simulink model "send_mmf"  (R2016a)
settings: Solver=FixedStepAuto  StartTime=0.0  StopTime=10.0  RelTol=1e-3
libraries: simulink x1, dspsigops x1, dspnetwork x1
settings Model: Creator=Florian Wachter  LastModifiedBy=Florian

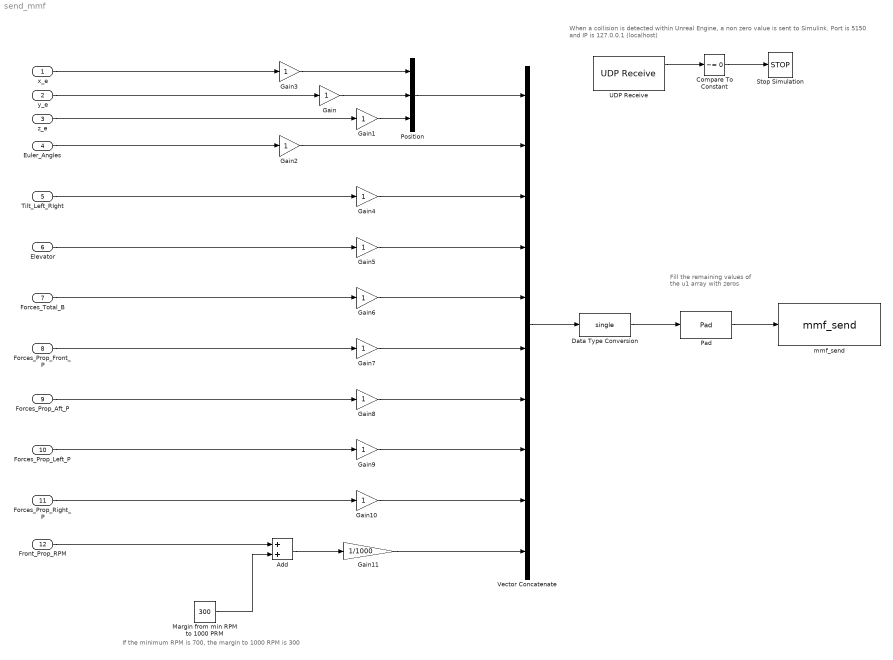
== system send_mmf ==
  note: If the minimum RPM is 700, the margin to 1000 RPM is 300
  note: Fill the remaining values of the u1 array with zeros
  note: When a collision is detected within Unreal Engine, a non zero value is sent to Simulink. Port is 5150 and IP is 127.0.0.1 (localhost)
  x_e : Inport
  y_e : Inport  Port=2
  z_e : Inport  Port=3
  Euler_Angles : Inport  Port=4
  Tilt_Left_RIght : Inport  Port=5
  Elevator : Inport  Port=6
  Forces_Total_B : Inport  Port=7
  Forces_Prop_Front_P : Inport  Port=8
  Forces_Prop_Aft_P : Inport  Port=9
  Forces_Prop_Left_P : Inport  Port=10
  Forces_Prop_Right_P : Inport  Port=11
  Front_Prop_RPM : Inport  Port=12
  Add : Sum
  Compare To Constant : simulink/Logic and Bit Operations/Compare To Constant  relop=~=  const=0  OutDataTypeStr=boolean
  Data Type Conversion : DataTypeConversion  OutMax=[100]  OutDataTypeStr=single
  Gain{,1..10} (11 alike) : Gain
  Gain11 : Gain  Gain=1/1000
  Margin from min RPM to 1000 PRM : Constant  Value=300
  Pad : dspsigops/Pad  padAlong=Rows  dimsToPad=1  valSrc=Specify via dialog  padVal=0  spec=Output size  padNumOutRowsSpecMethod=User-specified  numOutRows=1  padNumOutColsSpecMethod=User-specified  numOutCols=100  isVarDimsMode=off  padBeginning=0  padEnd=0  outSizeMode=User-specified  outSize=1  padSigAt=End  trunc_flag=None  roundingMode=Floor  overflowMode=off  truncOrWrapMode=Truncate  wrap_flag=None
  Position : Concatenate  NumInputs=3
  Stop Simulation : Stop
  UDP Receive : dspnetwork/UDP Receive  localURL='0.0.0.0'  localPort=5150  remoteURL='0.0.0.0'  remotePort=-1  recvBufferSize=1  dims=1  signalDatatype=uint8  isVarSize=off  showBlockingTime=off  blockingTime=0  sampletime=0.01
  Vector Concatenate : Concatenate  NumInputs=10
  mmf_send : S-Function  FunctionName=mmf_send  SFunctionDeploymentMode=off  EnableBusSupport=off  mask(Legacy Function){SFunctionSpec=void mmf_send(single u1[100]), ShowSpec=on}
      mask prompts: ShowSpec "Display function specification"
      mask help:
      | This block allows you to call the legacy functions specified by the following Legacy Code Tool definition:
      | def.SFunctionName = 'mmf_send';
      | def.OutputFcnSpec = 'void mmf_send(single u1[100])';
      | def.StartFcnSpec = 'mmf_init()';
      | def.TerminateFcnSpec = 'mmf_close()';
      | def.HeaderFiles = {'mmf_send_dll.h'};
      | def.HostLibFiles = {'mmf_send_dll.lib'};
      mask Help: <p>This block was generated automatically by the Legacy Code Tool. For detailed help on this tool, call<a href="matlab:legacy_code('help')"> legacy_code('help')</a>.</p>
      mask Callback ShowSpec:
      | if strcmp(get_param(gcbh, 'ShowSpec'), 'on')
      |   set_param(gcbh, 'MaskDisplay', sprintf('fprintf(''%s'');', get_param(gcbh, 'SFunctionSpec')));
      | else
      |   set_param(gcbh, 'MaskDisplay', sprintf('fprintf(''%s'');', get_param(gcbh, 'FunctionName')));
      | end
      mask Display: fprintf('void mmf_send(single u1[100])');
  wires:
  Data Type Conversion/1 -> Pad/1
  Vector Concatenate/1 -> Data Type Conversion/1
  Position/1 -> Vector Concatenate/1
  Pad/1 -> mmf_send/1
  Gain/1 -> Position/2
  Gain1/1 -> Position/3
  Gain3/1 -> Position/1
  x_e/1 -> Gain3/1
  y_e/1 -> Gain/1
  Euler_Angles/1 -> Gain2/1
  UDP Receive/1 -> Compare To Constant/1
  Compare To Constant/1 -> Stop Simulation/1
  z_e/1 -> Gain1/1
  Gain2/1 -> Vector Concatenate/2
  Tilt_Left_RIght/1 -> Gain4/1
  Gain4/1 -> Vector Concatenate/3
  Elevator/1 -> Gain5/1
  Gain5/1 -> Vector Concatenate/4
  Forces_Total_B/1 -> Gain6/1
  Gain6/1 -> Vector Concatenate/5
  Forces_Prop_Front_P/1 -> Gain7/1
  Gain7/1 -> Vector Concatenate/6
  Forces_Prop_Aft_P/1 -> Gain8/1
  Gain8/1 -> Vector Concatenate/7
  Forces_Prop_Left_P/1 -> Gain9/1
  Gain9/1 -> Vector Concatenate/8
  Forces_Prop_Right_P/1 -> Gain10/1
  Gain10/1 -> Vector Concatenate/9
  Gain11/1 -> Vector Concatenate/10
  Add/1 -> Gain11/1
  Front_Prop_RPM/1 -> Add/1
  Margin from min RPM to 1000 PRM/1 -> Add/2
